simulink model "autosar_swc_slfcns"  (R2022b)
settings: Solver=FixedStepDiscrete  StartTime=0.0  StopTime=10.0  FixedStep=1  RelTol=1e-3  EnableMultiTasking=on
PreLoadFcn:
  | Simulink.defineIntEnumType(...
  |  'ExampleErrorEnum', ...
  |  {'E_OK',  'E_NOT_OK', 'E_OVERFLOW', 'E_UNDERFLOW'}, ...
  |  [0, 1, 2, 3], ...
  |   'DefaultValue', 'E_OK', ...
  |  'HeaderFile', 'Rte_Type.h', ...
  |  'DataScope', 'Imported', ...
  |  'StorageType', 'uint8', ...
  |  'AddClassNameToEnumNames', false ...
  | );
  | 
  | Std_ReturnType = Simulink.AliasType;
  | Std_ReturnType.HeaderFile = 'Rte_Type.h';
  | Std_ReturnType.BaseType = 'uint8';
undefined symbols (not defined in the file): ExampleErrorEnum
libraries: simulink x1
settings Model: ModifiedByFormat=The MathWorks Inc.  Creator=The MathWorks, Inc.  LastModifiedBy=The MathWorks Inc.
settings SolverCC: AlgebraicLoopSolver=TrustRegion  MinimalZcImpactIntegration=on  MaxZcPerStep=1
settings DataIOCC: LimitDataPoints=on  SaveFormat=Array  SaveOutput=off  SaveTime=off  ReturnWorkspaceOutputs=off  SignalLoggingName=sigsOut
settings OptimizationCC: DefaultParameterBehavior=Inlined  UseDivisionForNetSlopeComputation=on  InlineInvariantSignals=on  EnhancedBackFolding=on  ExpressionDepthLimit=2147483647  StateBitsets=on  DataBitsets=on  ZeroExternalMemoryAtStartup=off  NoFixptDivByZeroProtection=on  EfficientFloat2IntCast=on  LifeSpan=1  EfficientTunableParamExpr=on
settings DebuggingCC: CheckExecutionContextPreStartOutputMsg=on  AllowSymbolicDim=off  StateNameClashWarn=warning  PregeneratedLibrarySubsystemCodeDiagnostic=none  StrictBusMsg=ErrorOnBusTreatedAsVector  SFUnexpectedBacktrackingDiag=warning  SFNoUnconditionalDefaultTransitionDiag=warning  SFExecutionAtInitializationDiag=none  SFMachineParentedDataDiag=warning  ArithmeticOperatorsInVariantConditions=warning
settings HardwareCC: TargetHWDeviceType=Generic->32-bit Embedded Processor
settings ModelReferenceCC: UpdateModelReferenceTargets=IfOutOfDate  EnableRefExpFcnMdlSchedulingChecks=on  PropagateSignalLabelsOutOfModel=off
settings SFSimCC: SimUseLocalCustomCode=off  MATLABDynamicMemAlloc=off  CustomCodeUndefinedFunction=UseInterfaceOnly
settings RTWCC: Description=AUTOSAR  SystemTargetFile=autosar.tlc  TLCOptions=-p0 -aWarnNonSaturatedBlocks=0  GenCodeOnly=on  TemplateMakefile=ert_default_tmf  GenerateReport=on  RTWVerbose=off  RTWUseLocalCustomCode=off  IncludeHyperlinkInReport=on  LaunchReport=on  GenerateTraceInfo=on  GenerateTraceReport=on  GenerateTraceReportSl=on  GenerateTraceReportSf=on  GenerateTraceReportEml=on  GenerateCodeMetricsReport=on  DLArmComputeVersion=19.05
settings CodeAppCC: ForceParamTrailComments=on  IgnoreCustomStorageClasses=off  SimulinkDataObjDesc=on  CustomSymbolStrGlobalVar=rt$N$M  CustomSymbolStrType=$N$M  CustomSymbolStrFcn=$N$M$F  CustomSymbolStrModelFcn=$N  CustomSymbolStrMacro=$N$M  InsertBlockDesc=on  StateflowObjectComments=on
settings STFCustomTargetCC: UtilityFuncGeneration=Shared location  ParMdlRefBuildCompliant=on  CompOptLevelCompliant=on  IncludeMdlTerminateFcn=off  CombineOutputUpdateFcns=on  SuppressErrorStatus=on  ERTCustomFileBanners=on  SupportNonFinite=off  SupportComplex=off  SupportContinuousTime=off  SupportNonInlinedSFcns=off  RemoveResetFunc=on  MATLABClassNameForMDSCustomization=Simulink.SoftwareTarget.ERTCustomization  CPPClassGenCompliant=on  AutosarCompliant=on  UseToolchainInfoCompliant=on  LookupTableObjectStructAxisOrder=2,1,3,4,...  LUTObjectStructOrderEvenSpacing=Size,Table,Breakpoints  SystemTargetFile=autosar.tlc
settings ERTTargetCC: UtilityFuncGeneration=Shared location  MultiwordLength=2048  ConcurrentExecutionCompliant=off  IncludeMdlTerminateFcn=off  SuppressErrorStatus=on  SupportNonFinite=off  SupportComplex=off  ModelStepFunctionPrototypeControlCompliant=off  AutosarCompliant=on  LookupTableObjectStructAxisOrder=2,1,3,4,...  LUTObjectStructOrderEvenSpacing=Size,Table,Breakpoints  InlinedParameterPlacement=NonHierarchical  ERTCustomFileTemplate=example_file_process.tlc  ConvertIfToSwitch=off  SuppressUnreachableDefaultCases=off
settings ConfigComp: CovMetricSettings=dw  CovSaveCumulativeToWorkspaceVar=on  CovSaveSingleToWorkspaceVar=on  CovExternalEMLEnable=off  CovSFcnEnable=off
settings SimscapeCC: SimscapeNormalizeSystem=off  SimscapeNominalValues={1, 'bar'; 1, 'cm^3/s'; 1, 'bar*kg/s'; 1, 'kJ/kg'; 1, 'kW'; };

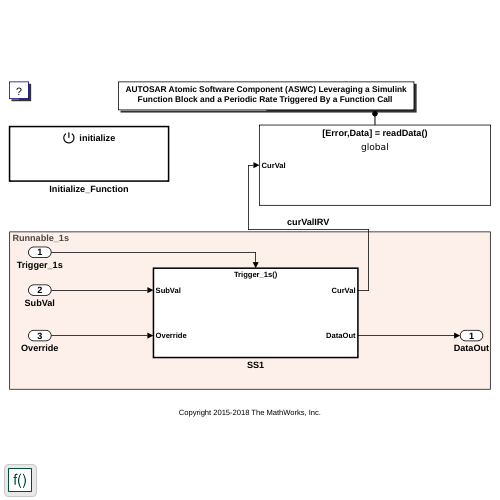
[thumbnail: Simulink's stored preview of the top-level diagram]
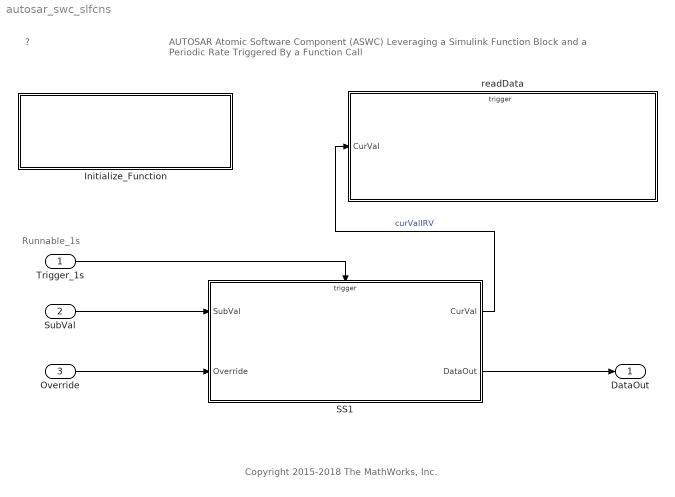
== system autosar_swc_slfcns ==
  note: Runnable_1s
  note: Copyright 2015-2018 The MathWorks, Inc.
  note: ?
  note: AUTOSAR Atomic Software Component (ASWC) Leveraging a Simulink Function Block and a Periodic Rate Triggered By a Function Call
  Trigger_1s : Inport  SampleTime=1  OutputFunctionCall=on
  SubVal : Inport  Port=2
  Override : Inport  Port=3
  Initialize_Function : Subsystem  TreatAsAtomicUnit=on
  SS1 : Subsystem  TreatAsAtomicUnit=on  RTWFcnName=foo
  readData : Subsystem  TreatAsAtomicUnit=on  RTWFcnName=foo
      settings: RTWSystemCode=Nonreusable function
  DataOut : Outport  InitialOutput=0  VectorParamsAs1DForOutWhenUnconnected=off
  wires:
  Trigger_1s/1 -> SS1/Trigger
  SS1/2(DataOut) -> DataOut/1
  SS1/1(CurVal) -> readData/1(CurVal)  "curValIRV"
  SubVal/1 -> SS1/1(SubVal)
  Override/1 -> SS1/2(Override)

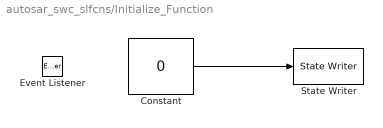
== system autosar_swc_slfcns/Initialize_Function ==
  Constant : Constant  DisableCoverage=on  Value=0  OutDataTypeStr=uint16
  Event Listener : EventListener  DisableCoverage=on  EventName=reset
  State Writer : StateWriter  DisableCoverage=on  StateOwnerBlock=../../SS1/RollingCounter/UnitDelay
  wires:
  Constant/1 -> State Writer/1

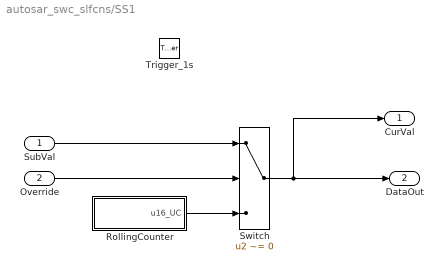
== system autosar_swc_slfcns/SS1 ==
  SubVal : Inport
  Override : Inport  Port=2
  Trigger_1s : TriggerPort  TriggerType=function-call  VariantControl=Variant  SampleTimeType=periodic
  RollingCounter : Subsystem  RTWFcnName=foo
  Switch : Switch  Criteria=u2 ~= 0  SaturateOnIntegerOverflow=off  InputSameDT=off
  CurVal : Outport  VectorParamsAs1DForOutWhenUnconnected=off
  DataOut : Outport  Port=2  OutDataTypeStr=uint16  InitialOutput=0  VectorParamsAs1DForOutWhenUnconnected=off
  wires:
  Override/1 -> Switch/2
  Switch/1 -> CurVal/1, DataOut/1
  SubVal/1 -> Switch/1
  RollingCounter/1(u16_UC) -> Switch/3

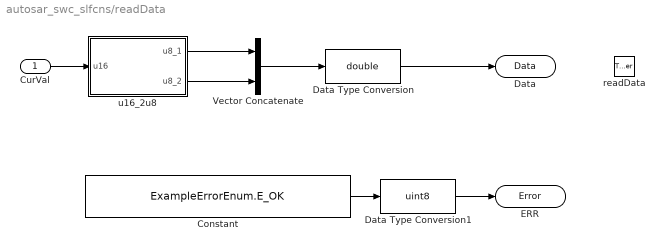
== system autosar_swc_slfcns/readData ==
  CurVal : Inport
  readData : TriggerPort  TriggerType=function-call  IsSimulinkFunction=on  FunctionName=readData  VariantControl=Variant  PortDimensions=1
  Constant : Constant  Value=ExampleErrorEnum.E_OK
  Data Type Conversion : DataTypeConversion  OutDataTypeStr=double  SaturateOnIntegerOverflow=off  RndMeth=Floor
  Data Type Conversion1 : DataTypeConversion  OutDataTypeStr=uint8  SaturateOnIntegerOverflow=off  RndMeth=Floor
  Vector Concatenate : Concatenate
  u16_2u8 : Stateflow chart  TreatAsAtomicUnit=on
  ERR : ArgOut  OutDataTypeStr=Std_ReturnType  ArgumentName=Error
  Data : ArgOut  Port=2  PortDimensions=2  ArgumentName=Data
  wires:
  u16_2u8/2(u8_2) -> Vector Concatenate/2
  u16_2u8/1(u8_1) -> Vector Concatenate/1
  CurVal/1 -> u16_2u8/1(u16)
  Vector Concatenate/1 -> Data Type Conversion/1
  Data Type Conversion/1 -> Data/1
  Constant/1 -> Data Type Conversion1/1
  Data Type Conversion1/1 -> ERR/1

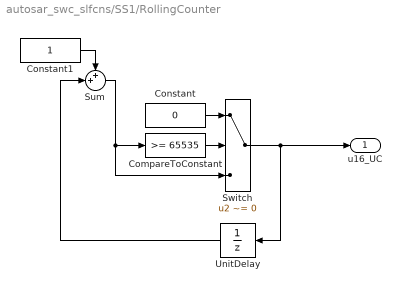
== system autosar_swc_slfcns/SS1/RollingCounter ==
  CompareToConstant : simulink/Logic and Bit Operations/Compare To Constant  relop=>=  const=65535  OutDataTypeStr=boolean  ZeroCross=off
  Constant : Constant  Value=0  OutDataTypeStr=uint16
  Constant1 : Constant  OutDataTypeStr=uint16
  Sum : Sum  Inputs=++|
  Switch : Switch  Criteria=u2 ~= 0  SaturateOnIntegerOverflow=off  InputSameDT=off
  UnitDelay : UnitDelay  SampleTime=-1  HasFrameUpgradeWarning=on
  u16_UC : Outport  OutDataTypeStr=uint16  VectorParamsAs1DForOutWhenUnconnected=off
  wires:
  Sum/1 -> Switch/3, CompareToConstant/1
  CompareToConstant/1 -> Switch/2
  Constant/1 -> Switch/1
  Switch/1 -> u16_UC/1, UnitDelay/1
  Constant1/1 -> Sum/1
  UnitDelay/1 -> Sum/2

== stateflow chart autosar_swc_slfcns/readData/u16_2u8 ==
  (default) -> (junction 1)
  (junction 1) -> (junction 2) : {u8_1 = u16;
      | u8_2 = u16 >> 8;}
  data: u16 input uint16; u8_1 output uint8; u8_2 output uint8
